simulink model "arm_sim_following"  (R2022a)
settings: Solver=ode4  StartTime=0.0  StopTime=3  FixedStep=0.001  RelTol=1e-3
undefined symbols (not defined in the file): A, B, C, dc, H, K, rc, x0
settings Model: Creator=kawata  LastModifiedBy=kawata
settings SolverCC: AlgebraicLoopSolver=TrustRegion
settings DataIOCC: ReturnWorkspaceOutputs=off
settings DebuggingCC: UnconnectedInputMsg=warning  UnconnectedOutputMsg=warning  UnconnectedLineMsg=warning  SFMachineParentedDataDiag=warning  ArithmeticOperatorsInVariantConditions=warning
settings SFSimCC: SimUseLocalCustomCode=off  CustomCodeUndefinedFunction=UseInterfaceOnly
settings RTWCC: RTWUseLocalCustomCode=off

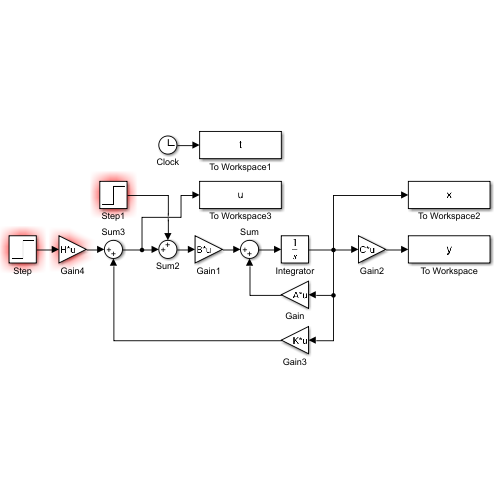
[thumbnail: Simulink's stored preview of the top-level diagram]
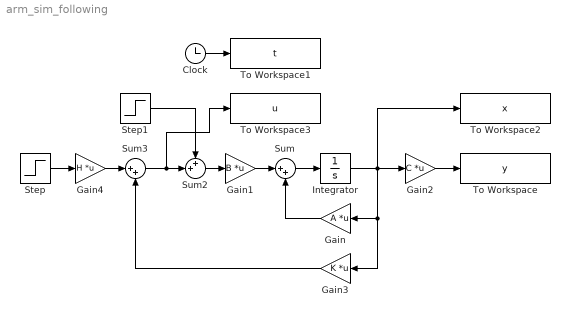
== system arm_sim_following ==
  Clock : Clock
  Gain : Gain  Gain=A  Multiplication=Matrix(K*u)
  Gain1 : Gain  Gain=B  Multiplication=Matrix(K*u)
  Gain2 : Gain  Gain=C  Multiplication=Matrix(K*u)
  Gain3 : Gain  Gain=K  Multiplication=Matrix(K*u)
  Gain4 : Gain  Gain=H  Multiplication=Matrix(K*u)
  Integrator : Integrator  InitialCondition=x0
  Step : Step  Time=0  After=rc  SampleTime=0
  Step1 : Step  Time=1.5  After=dc  SampleTime=0
  Sum : Sum  Inputs=|++
  Sum2 : Sum  Inputs=++|
  Sum3 : Sum  Inputs=|++
  To Workspace : ToWorkspace  VariableName=y  SampleTime=-1
  To Workspace1 : ToWorkspace  VariableName=t  SampleTime=-1
  To Workspace2 : ToWorkspace  VariableName=x  SampleTime=-1
  To Workspace3 : ToWorkspace  VariableName=u  SampleTime=-1
  wires:
  Clock/1 -> To Workspace1/1
  Sum3/1 -> To Workspace3/1, Sum2/2
  Step/1 -> Gain4/1
  Sum/1 -> Integrator/1
  Gain3/1 -> Sum3/2
  Step1/1 -> Sum2/1
  Integrator/1 -> To Workspace2/1, Gain3/1, Gain/1, Gain2/1
  Gain/1 -> Sum/2
  Gain1/1 -> Sum/1
  Gain4/1 -> Sum3/1
  Sum2/1 -> Gain1/1
  Gain2/1 -> To Workspace/1
